simulink model "thalamicIsolated"  (Simulink 9.3)
settings: Solver=ode4  StartTime=0.0  StopTime=60  FixedStep=.004  RelTol=1e-3  EnableMultiTasking=on
Description:
  | Author: Ali Najmaldin
settings Model: Creator=Author: Ali Najmaldin  LastModifiedBy=alinajmaldin  SimulationMode=accelerator
settings DataIOCC: SaveOutput=off  SignalLogging=off  SaveTime=off
settings OptimizationCC: ExpressionDepthLimit=2147483647
settings DebuggingCC: SaveWithParameterizedLinksMsg=none  SolverPrmCheckMsg=warning  InheritedTsInSrcMsg=none  ModelReferenceDataLoggingMessage=none  StateNameClashWarn=warning
settings SFSimCC: SimParseCustomCode=off

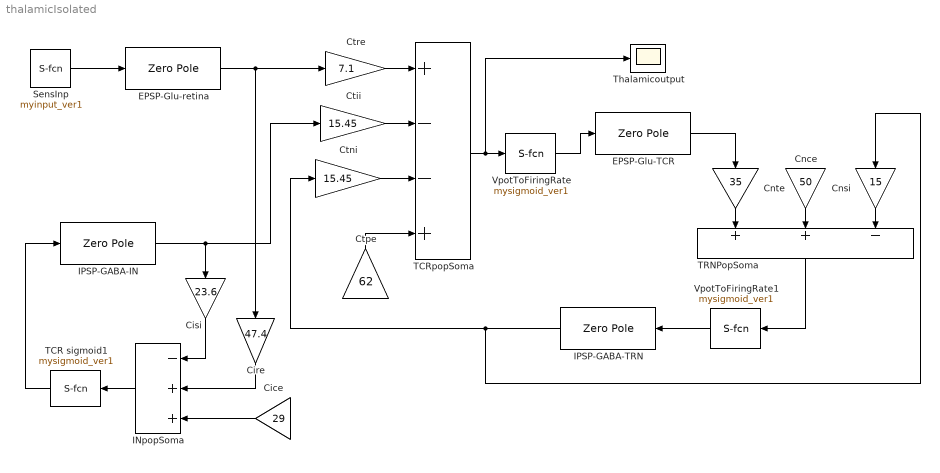
== system thalamicIsolated ==
  Cice : Gain  Gain=29
  Cire : Gain  Gain=47.4
  Cisi : Gain  Gain=23.6
  Cnce : Gain  Gain=50
  Cnsi : Gain  Gain=15
  Cnte : Gain  Gain=35
  Ctii : Gain  Gain=15.45
  Ctni : Gain  Gain=15.45
  Ctpe : Gain  Gain=62
  Ctre : Gain  Gain=7.1
  EPSP-Glu-TCR : ZeroPole  Zeros=[]  Poles=[-100 -100]  Gain=[0.00325*100]
  EPSP-Glu-retina : ZeroPole  Zeros=[]  Poles=[-100 -100]  Gain=[0.00325*100]
  INpopSoma : Sum  Inputs=-++  CollapseMode=Specified dimension  CollapseDim=4
  IPSP-GABA-IN : ZeroPole  Zeros=[]  Poles=[-40 -40]  Gain=[0.022*40]
  IPSP-GABA-TRN : ZeroPole  Zeros=[]  Poles=[-40 -40]  Gain=[0.022*40]
  SensInp : M-S-Function  Description=|  FunctionName=myinput_ver1  Parameters=11,5,60000,1
      | Input to the model with or without noise. The order of input parameters in the Dialog box is:                      
      | mean, standard deviation, length of signal,flag,constant.                                                          
      | If flag is 0, the input is a constant devoid of any noise. However, if flag is 1, the noise is added to the signal.
      mask Display: plot(312+randn(1,25))
  TCR sigmoid1 : M-S-Function  FunctionName=mysigmoid_ver1  Parameters=2.5,560,0.006
      mask Display: plot(1./(1+exp(-0.75.*([1:25]-12))))
  TCRpopSoma : Sum  Inputs=+--+  CollapseMode=Specified dimension  CollapseDim=4
  TRNPopSoma : Sum  Inputs=++-  CollapseMode=Specified dimension  CollapseDim=4
  Thalamicoutput : Scope
  VpotToFiringRate : M-S-Function  FunctionName=mysigmoid_ver1  Parameters=2.5,560,0.006
      mask Display: plot(1./(1+exp(-0.75.*([1:25]-12))))
  VpotToFiringRate1 : M-S-Function  FunctionName=mysigmoid_ver1  Parameters=2.5,560,0.006
      mask Display: plot(1./(1+exp(-0.75.*([1:25]-12))))
  wires:
  Ctre/1 -> TCRpopSoma/1
  SensInp/1 -> EPSP-Glu-retina/1
  EPSP-Glu-retina/1 -> Ctre/1, Cire/1
  TCRpopSoma/1 -> VpotToFiringRate/1, Thalamicoutput/1
  INpopSoma/1 -> TCR sigmoid1/1
  Cire/1 -> INpopSoma/2
  TCR sigmoid1/1 -> IPSP-GABA-IN/1
  IPSP-GABA-IN/1 -> Ctii/1, Cisi/1
  TRNPopSoma/1 -> VpotToFiringRate1/1
  VpotToFiringRate/1 -> EPSP-Glu-TCR/1
  Cnte/1 -> TRNPopSoma/1
  VpotToFiringRate1/1 -> IPSP-GABA-TRN/1
  IPSP-GABA-TRN/1 -> Ctni/1, Cnsi/1
  Cnce/1 -> TRNPopSoma/2
  Ctii/1 -> TCRpopSoma/2
  Ctni/1 -> TCRpopSoma/3
  Ctpe/1 -> TCRpopSoma/4
  Cisi/1 -> INpopSoma/1
  Cice/1 -> INpopSoma/3
  Cnsi/1 -> TRNPopSoma/3
  EPSP-Glu-TCR/1 -> Cnte/1
